simulink model "Testing_Response"  (R2021a)
settings: Solver=VariableStepAuto  StartTime=0.0  StopTime=10.0  RelTol=1e-3
libraries: simulink_extras x8
settings Model: Creator=Bishoy Zaky  LastModifiedBy=Bishoy Zaky

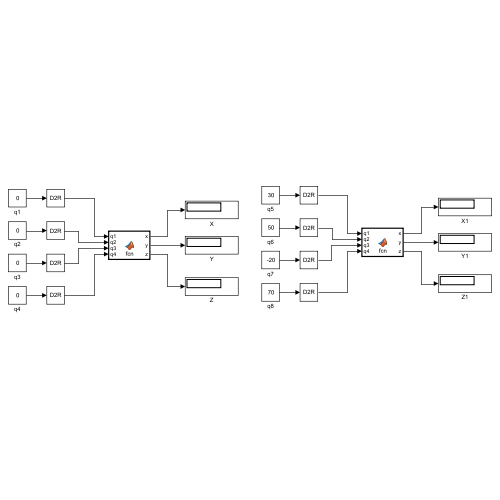
[thumbnail: Simulink's stored preview of the top-level diagram]
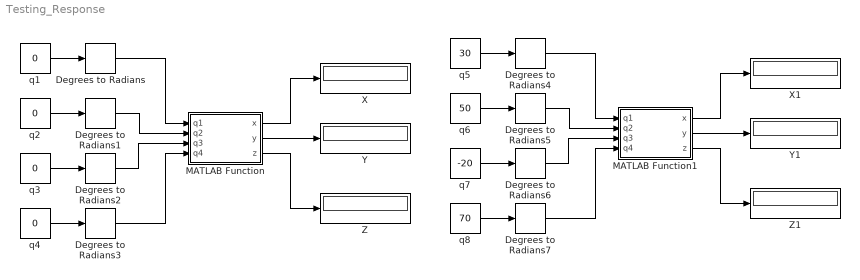
== system Testing_Response ==
  Degrees to Radians{,1..7} (8 alike) : simulink_extras/Transformations/Degrees to Radians
  MATLAB Function : MATLAB Function  TreatAsAtomicUnit=on
  MATLAB Function1 : MATLAB Function  TreatAsAtomicUnit=on
  X : Display
  X1 : Display
  Y : Display
  Y1 : Display
  Z : Display
  Z1 : Display
  q{1..4} (4 alike) : Constant  Value=0
  q5 : Constant  Value=30
  q6 : Constant  Value=50
  q7 : Constant  Value=-20
  q8 : Constant  Value=70
  wires:
  q1/1 -> Degrees to Radians/1
  q2/1 -> Degrees to Radians1/1
  q3/1 -> Degrees to Radians2/1
  q4/1 -> Degrees to Radians3/1
  Degrees to Radians/1 -> MATLAB Function/1(q1)
  Degrees to Radians1/1 -> MATLAB Function/2(q2)
  Degrees to Radians2/1 -> MATLAB Function/3(q3)
  Degrees to Radians3/1 -> MATLAB Function/4(q4)
  MATLAB Function/1(x) -> X/1
  MATLAB Function/2(y) -> Y/1
  MATLAB Function/3(z) -> Z/1
  MATLAB Function1/1(x) -> X1/1
  q5/1 -> Degrees to Radians4/1
  q6/1 -> Degrees to Radians5/1
  MATLAB Function1/2(y) -> Y1/1
  Degrees to Radians4/1 -> MATLAB Function1/1(q1)
  Degrees to Radians7/1 -> MATLAB Function1/4(q4)
  Degrees to Radians5/1 -> MATLAB Function1/2(q2)
  Degrees to Radians6/1 -> MATLAB Function1/3(q3)
  q8/1 -> Degrees to Radians7/1
  q7/1 -> Degrees to Radians6/1
  MATLAB Function1/3(z) -> Z1/1

== matlab function Testing_Response/MATLAB Function1 ==
  data: x output; q1 input; y output; q2 input; q3 input; q4 input; z output
function [x,y,z] = fcn(q1,q2,q3,q4)
x = 24.63*sin(q1) - 5.6e-17*cos(q3)*(3.25e+18*cos(q2 + 1.571)*cos(q1)...
    - 199.0*sin(q2 + 1.571)*sin(q1)) + 5.6e-17*sin(q3)*(199.0*cos(q2 + 1.571)*sin(q1)...
    + 3.25e+18*sin(q2 + 1.571)*cos(q1)) - 2.0e-19*cos(q4 - 1.233)*...
    (2.637e+20*cos(q2 - 1.0*q1 + q3 + 1.571) + 2.637e+20*cos(q1 + q2 + q3 + 1.571))...
    + 2.0e-19*sin(q4 - 1.233)*(2.637e+20*sin(q2 - 1.0*q1 + q3 + 1.571) + 2.637e+20*...
    sin(q1 + q2 + q3 + 1.571)) - 182.0*cos(q2 + 1.571)*cos(q1) + 1.114e-14*sin(q2 + 1.571)*sin(q1);
y = 2.0e-19*sin(q4 - 1.233)*(2.637e+20*cos(q2 - 1.0*q1 + q3 + 1.571)...
    - 2.637e+20*cos(q1 + q2 + q3 + 1.571)) - 5.6e-17*cos(q3)*(3.25e+18*cos(q2 + 1.571)*sin(q1)...
    + 199.0*sin(q2 + 1.571)*cos(q1)) - 5.6e-17*sin(q3)*(199.0*cos(q2 + 1.571)*cos(q1) - 3.25e+18*...
    sin(q2 + 1.571)*sin(q1)) - 24.63*cos(q1) + 2.0e-19*cos(q4 - 1.233)*(2.637e+20*...
    sin(q2 - 1.0*q1 + q3 + 1.571) - 2.637e+20*sin(q1 + q2 + q3 + 1.571)) - 182.0*...
    cos(q2 + 1.571)*sin(q1) - 1.114e-14*sin(q2 + 1.571)*cos(q1);
z = - 182.0*sin(q2 + q3 + 1.571) - 105.5*sin(q2 + q3 + q4 + 0.3382) - 182.0*cos(q2 + 3.673e-6) - 42.5;

== matlab function Testing_Response/MATLAB Function ==
  data: x output; q1 input; y output; q2 input; q3 input; q4 input; z output
function [x,y,z] = fcn(q1,q2,q3,q4)
x = 24.63*sin(q1) - 5.6e-17*cos(q3)*(3.25e+18*cos(q2 + 1.571)*cos(q1)...
    - 199.0*sin(q2 + 1.571)*sin(q1)) + 5.6e-17*sin(q3)*(199.0*cos(q2 + 1.571)*sin(q1)...
    + 3.25e+18*sin(q2 + 1.571)*cos(q1)) - 2.0e-19*cos(q4 - 1.233)*...
    (2.637e+20*cos(q2 - 1.0*q1 + q3 + 1.571) + 2.637e+20*cos(q1 + q2 + q3 + 1.571))...
    + 2.0e-19*sin(q4 - 1.233)*(2.637e+20*sin(q2 - 1.0*q1 + q3 + 1.571) + 2.637e+20*...
    sin(q1 + q2 + q3 + 1.571)) - 182.0*cos(q2 + 1.571)*cos(q1) + 1.114e-14*sin(q2 + 1.571)*sin(q1);
y = 2.0e-19*sin(q4 - 1.233)*(2.637e+20*cos(q2 - 1.0*q1 + q3 + 1.571)...
    - 2.637e+20*cos(q1 + q2 + q3 + 1.571)) - 5.6e-17*cos(q3)*(3.25e+18*cos(q2 + 1.571)*sin(q1)...
    + 199.0*sin(q2 + 1.571)*cos(q1)) - 5.6e-17*sin(q3)*(199.0*cos(q2 + 1.571)*cos(q1) - 3.25e+18*...
    sin(q2 + 1.571)*sin(q1)) - 24.63*cos(q1) + 2.0e-19*cos(q4 - 1.233)*(2.637e+20*...
    sin(q2 - 1.0*q1 + q3 + 1.571) - 2.637e+20*sin(q1 + q2 + q3 + 1.571)) - 182.0*...
    cos(q2 + 1.571)*sin(q1) - 1.114e-14*sin(q2 + 1.571)*cos(q1);
z = - 182.0*sin(q2 + q3 + 1.571) - 105.5*sin(q2 + q3 + q4 + 0.3382) - 182.0*cos(q2 + 3.673e-6) - 42.5;
